simulink model "Model_2ndPoint"  (R2023b)
settings: Solver=VariableStepAuto  StartTime=0.0  StopTime=H  RelTol=1e-3
values from neighbouring files (symbols this model uses):
  C_f = c_f*m_f    (= 360000)    [init.m]
  C_f_2 = c_f_2*m_f_2    (= 360000)    [init.m]
  C_f_3 = c_f_3*m_f_3    (= 240000)    [init.m]
  C_f_4 = c_f_4*m_f_4    (= 480000)    [init.m]
  k_fc = barK_fc*s_c    (= 570)    [init.m]
  q_s = barK_fc * a    (= 5.529)    [init.m]
  theta0_f = 280    [init.m]
  Ts = 5    [init.m]
  var_wf = 1    [init.m]
settings Model: Creator=adil2  LastModifiedBy=adil2

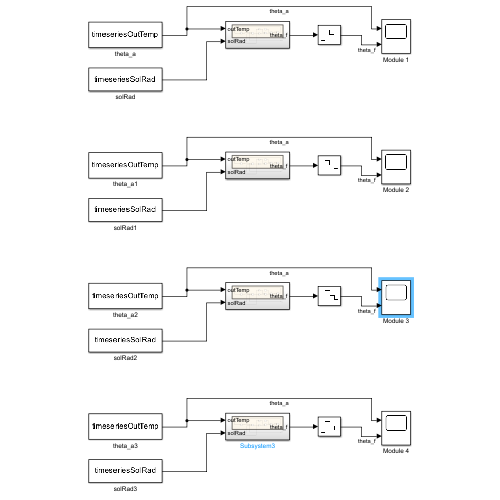
[thumbnail: Simulink's stored preview of the top-level diagram]
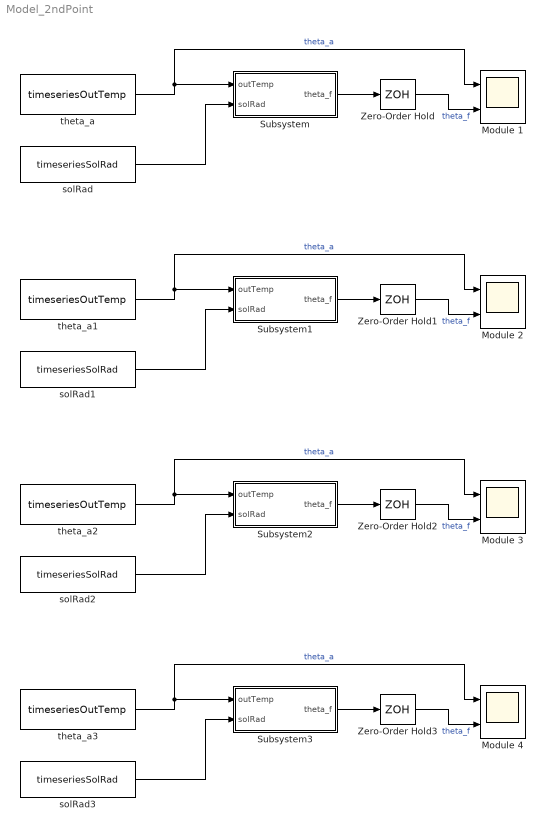
== system Model_2ndPoint ==
  Module {1..4} (4 alike) : Scope  NumInputPorts=2
  Subsystem : Subsystem
  Subsystem1 : Subsystem
  Subsystem2 : Subsystem
  Subsystem3 : Subsystem
  Zero-Order Hold{,1..3} (4 alike) : ZeroOrderHold  SampleTime=Ts
  solRad{,1..3} (4 alike) : FromWorkspace  VariableName=timeseriesSolRad
  theta_a{,1..3} (4 alike) : FromWorkspace  VariableName=timeseriesOutTemp  SampleTime=Ts
  wires:
  theta_a/1 -> Module 1/1, Subsystem/1(outTemp)  "theta_a"
  Subsystem/1(theta_f) -> Zero-Order Hold/1
  Zero-Order Hold/1 -> Module 1/2  "theta_f"
  solRad/1 -> Subsystem/2(solRad)
  Zero-Order Hold1/1 -> Module 2/2  "theta_f"
  theta_a1/1 -> Module 2/1, Subsystem1/1(outTemp)  "theta_a"
  Subsystem1/1(theta_f) -> Zero-Order Hold1/1
  solRad1/1 -> Subsystem1/2(solRad)
  Zero-Order Hold2/1 -> Module 3/2  "theta_f"
  theta_a2/1 -> Module 3/1, Subsystem2/1(outTemp)  "theta_a"
  Subsystem2/1(theta_f) -> Zero-Order Hold2/1
  solRad2/1 -> Subsystem2/2(solRad)
  theta_a3/1 -> Module 4/1, Subsystem3/1(outTemp)  "theta_a"
  Zero-Order Hold3/1 -> Module 4/2  "theta_f"
  Subsystem3/1(theta_f) -> Zero-Order Hold3/1
  solRad3/1 -> Subsystem3/2(solRad)

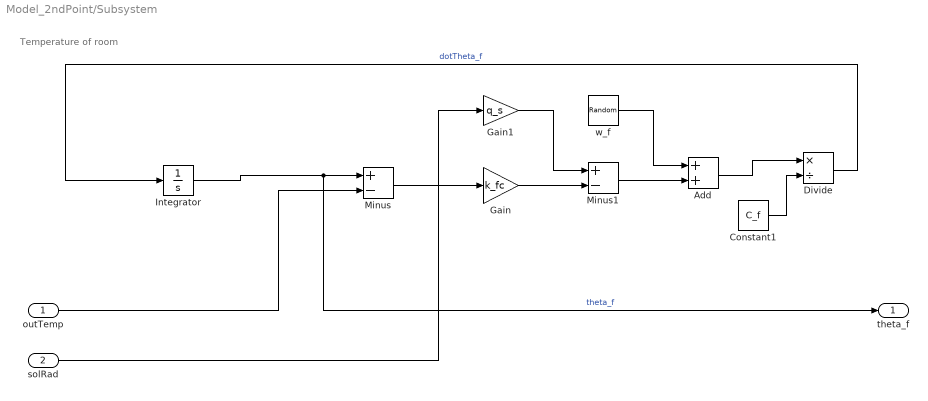
== system Model_2ndPoint/Subsystem ==
  note: Temperature of room
  outTemp : Inport
  solRad : Inport  Port=2
  Add : Sum
  Constant1 : Constant  Value=C_f
  Divide : Product  Inputs=*/
  Gain : Gain  Gain=k_fc
  Gain1 : Gain  Gain=q_s
  Integrator : Integrator  InitialCondition=theta0_f
  Minus : Sum  Inputs=+-
  Minus1 : Sum  Inputs=+-
  w_f : RandomNumber  Variance=var_wf  SampleTime=Ts
  theta_f : Outport
  wires:
  outTemp/1 -> Minus/2
  Integrator/1 -> theta_f/1, Minus/1  "theta_f"
  Minus/1 -> Gain/1
  Constant1/1 -> Divide/2
  Divide/1 -> Integrator/1  "dotTheta_f"
  Gain/1 -> Minus1/2
  Minus1/1 -> Add/2
  w_f/1 -> Add/1
  Add/1 -> Divide/1
  solRad/1 -> Gain1/1
  Gain1/1 -> Minus1/1

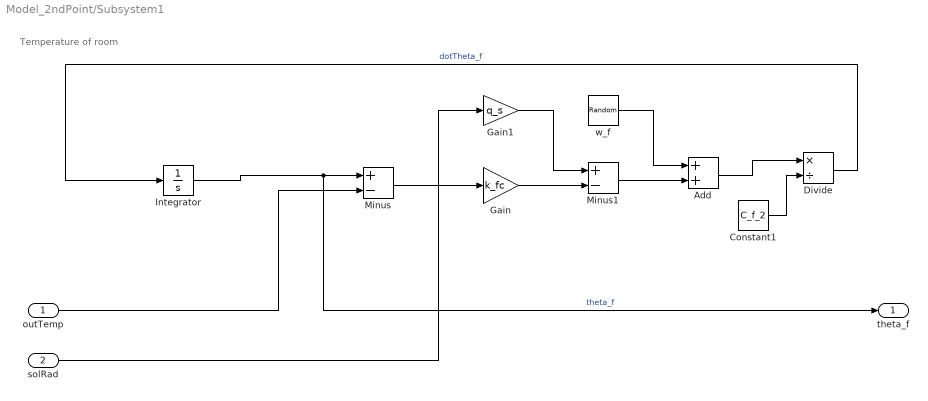
== system Model_2ndPoint/Subsystem1 ==
  note: Temperature of room
  outTemp : Inport
  solRad : Inport  Port=2
  Add : Sum
  Constant1 : Constant  Value=C_f_2
  Divide : Product  Inputs=*/
  Gain : Gain  Gain=k_fc
  Gain1 : Gain  Gain=q_s
  Integrator : Integrator  InitialCondition=theta0_f
  Minus : Sum  Inputs=+-
  Minus1 : Sum  Inputs=+-
  w_f : RandomNumber  Variance=var_wf  SampleTime=Ts
  theta_f : Outport
  wires:
  outTemp/1 -> Minus/2
  Integrator/1 -> theta_f/1, Minus/1  "theta_f"
  Minus/1 -> Gain/1
  Constant1/1 -> Divide/2
  Divide/1 -> Integrator/1  "dotTheta_f"
  Gain/1 -> Minus1/2
  Minus1/1 -> Add/2
  w_f/1 -> Add/1
  Add/1 -> Divide/1
  solRad/1 -> Gain1/1
  Gain1/1 -> Minus1/1

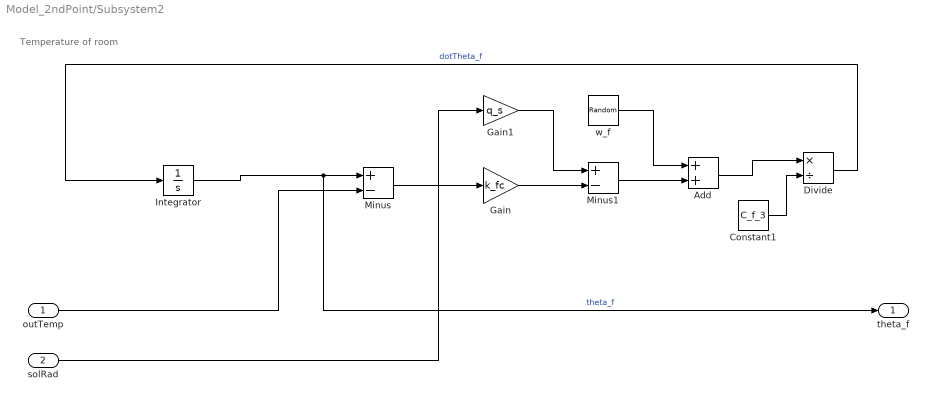
== system Model_2ndPoint/Subsystem2 ==
  note: Temperature of room
  outTemp : Inport
  solRad : Inport  Port=2
  Add : Sum
  Constant1 : Constant  Value=C_f_3
  Divide : Product  Inputs=*/
  Gain : Gain  Gain=k_fc
  Gain1 : Gain  Gain=q_s
  Integrator : Integrator  InitialCondition=theta0_f
  Minus : Sum  Inputs=+-
  Minus1 : Sum  Inputs=+-
  w_f : RandomNumber  Variance=var_wf  SampleTime=Ts
  theta_f : Outport
  wires:
  outTemp/1 -> Minus/2
  Integrator/1 -> theta_f/1, Minus/1  "theta_f"
  Minus/1 -> Gain/1
  Constant1/1 -> Divide/2
  Divide/1 -> Integrator/1  "dotTheta_f"
  Gain/1 -> Minus1/2
  Minus1/1 -> Add/2
  w_f/1 -> Add/1
  Add/1 -> Divide/1
  solRad/1 -> Gain1/1
  Gain1/1 -> Minus1/1

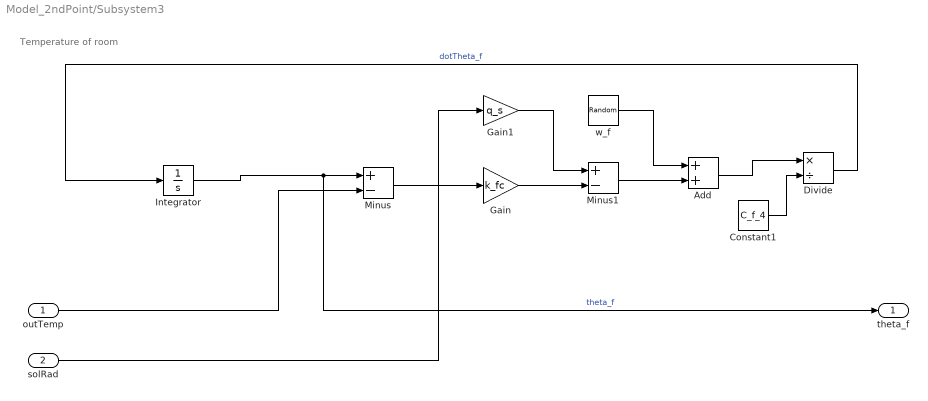
== system Model_2ndPoint/Subsystem3 ==
  note: Temperature of room
  outTemp : Inport
  solRad : Inport  Port=2
  Add : Sum
  Constant1 : Constant  Value=C_f_4
  Divide : Product  Inputs=*/
  Gain : Gain  Gain=k_fc
  Gain1 : Gain  Gain=q_s
  Integrator : Integrator  InitialCondition=theta0_f
  Minus : Sum  Inputs=+-
  Minus1 : Sum  Inputs=+-
  w_f : RandomNumber  Variance=var_wf  SampleTime=Ts
  theta_f : Outport
  wires:
  outTemp/1 -> Minus/2
  Integrator/1 -> theta_f/1, Minus/1  "theta_f"
  Minus/1 -> Gain/1
  Constant1/1 -> Divide/2
  Divide/1 -> Integrator/1  "dotTheta_f"
  Gain/1 -> Minus1/2
  Minus1/1 -> Add/2
  w_f/1 -> Add/1
  Add/1 -> Divide/1
  solRad/1 -> Gain1/1
  Gain1/1 -> Minus1/1
